simulink subsystem "Liear accleration model"  (R2024a)
settings: Solver=VariableStepAuto  StartTime=0.0  StopTime=10.0  RelTol=1e-3
libraries: autolibshared x6
(part 1 of 4)
settings Model: Creator=Lenovo  LastModifiedBy=Lenovo

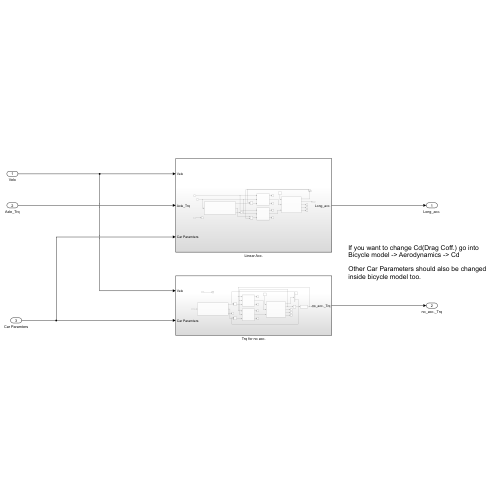
[thumbnail: Simulink's stored preview of the top-level diagram]
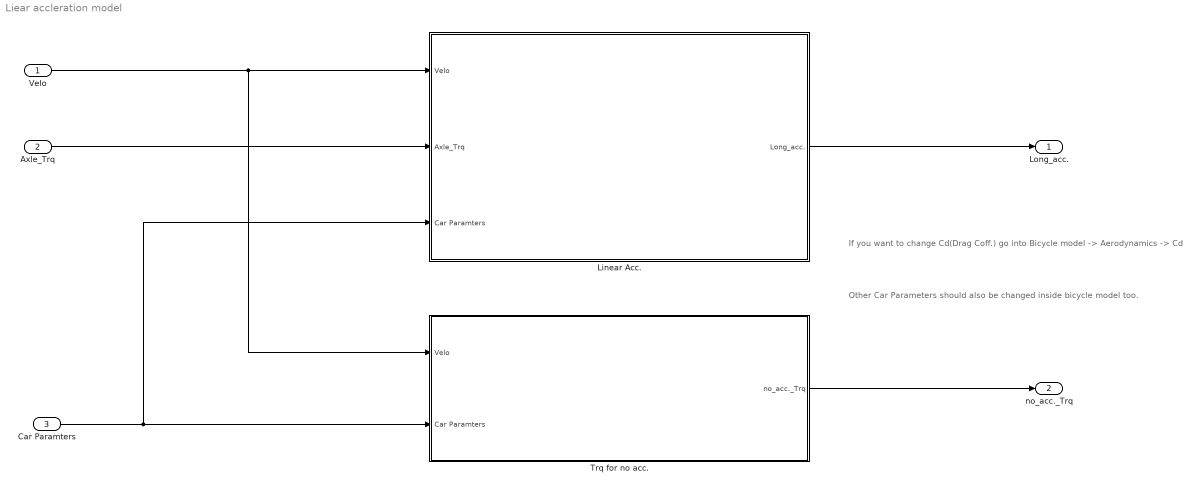
== system Liear accleration model ==
  note: If you want to change Cd(Drag Coff.) go into Bicycle model -> Aerodynamics -> Cd
  note: Other Car Parameters should also be changed inside bicycle model too.
  Velo : Inport
  Axle_Trq : Inport  Port=2
  Car Paramters : Inport  Port=3
  Linear Acc. : Subsystem
  Trq for no acc. : Subsystem
  Long_acc. : Outport
  no_acc._Trq : Outport  Port=2
  wires:
  Linear Acc./1(Long_acc.) -> Long_acc./1
  Trq for no acc./1(no_acc._Trq) -> no_acc._Trq/1
  Velo/1 -> Linear Acc./1(Velo), Trq for no acc./1(Velo)
  Axle_Trq/1 -> Linear Acc./2(Axle_Trq)
  Car Paramters/1 -> Trq for no acc./2(Car Paramters), Linear Acc./3(Car Paramters)
